simulink model "Subsystem"  (R2020b)
settings: Solver=FixedStepAuto  StartTime=0.0  StopTime=10.0  FixedStep=0.2  RelTol=1e-3
settings Model: Creator=ANUJA  LastModifiedBy=ANUJA
settings DataIOCC: SaveOutput=off  SaveTime=off

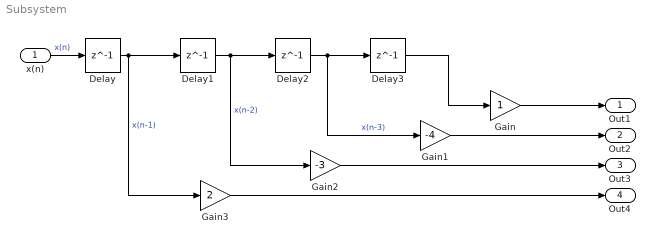
== system Subsystem ==
  x(n) : Inport  OutDataTypeStr=double  PortDimensions=1  SampleTime=[0,1]
  Delay{,1..3} (4 alike) : Delay  DelayLength=1  InitialCondition=0
  Gain : Gain
  Gain1 : Gain  Gain=-4
  Gain2 : Gain  Gain=-3
  Gain3 : Gain  Gain=2
  Out1 : Outport  OutDataTypeStr=double  PortDimensions=1  SampleTime=[0.20000000000000001,0]
  Out2 : Outport  Port=2  OutDataTypeStr=double  PortDimensions=1  SampleTime=[0.20000000000000001,0]
  Out3 : Outport  Port=3  OutDataTypeStr=double  PortDimensions=1  SampleTime=[0.20000000000000001,0]
  Out4 : Outport  Port=4  OutDataTypeStr=double  PortDimensions=1  SampleTime=[0.20000000000000001,0]
  wires:
  Gain3/1 -> Out4/1
  Delay1/1 -> Delay2/1, Gain2/1  "x(n-2)"
  Delay/1 -> Delay1/1, Gain3/1  "x(n-1)"
  Delay3/1 -> Gain/1
  Gain2/1 -> Out3/1
  Delay2/1 -> Gain1/1, Delay3/1  "x(n-3)"
  x(n)/1 -> Delay/1  "x(n)"
  Gain/1 -> Out1/1
  Gain1/1 -> Out2/1
